simulink model "ej"  (R2017b)
settings: Solver=VariableStepAuto  StartTime=0.0  StopTime=10.0  RelTol=1e-3
settings Model: Creator=Sofia  LastModifiedBy=Sofia

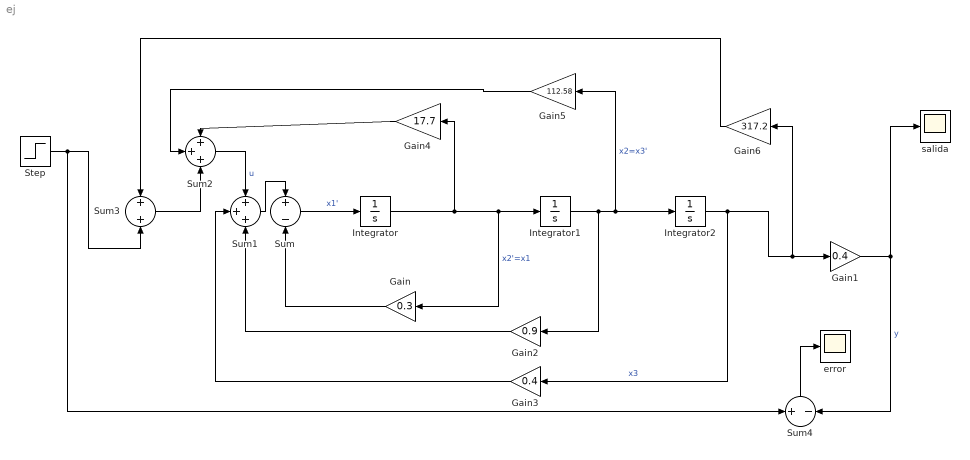
== system ej ==
  Gain : Gain  Gain=0.3
  Gain1 : Gain  Gain=0.4
  Gain2 : Gain  Gain=0.9
  Gain3 : Gain  Gain=0.4
  Gain4 : Gain  Gain=17.7
  Gain5 : Gain  Gain=112.58
  Gain6 : Gain  Gain=317.2
  Integrator : Integrator
  Integrator1 : Integrator
  Integrator2 : Integrator
  Step : Step  SampleTime=0
  Sum : Sum  Inputs=+-
  Sum1 : Sum  Inputs=+++
  Sum2 : Sum  Inputs=+++
  Sum3 : Sum
  Sum4 : Sum  Inputs=+-
  error : Scope
  salida : Scope
  wires:
  Sum/1 -> Integrator/1  "x1'"
  Sum1/1 -> Sum/1
  Integrator/1 -> Gain4/1, Integrator1/1, Gain/1  "x2'=x1"
  Gain/1 -> Sum/2
  Integrator1/1 -> Gain2/1, Gain5/1, Integrator2/1  "x2=x3'"
  Integrator2/1 -> Gain3/1, Gain6/1, Gain1/1  "x3"
  Gain1/1 -> Sum4/2, salida/1  "y"
  Sum2/1 -> Sum1/1  "u"
  Gain2/1 -> Sum1/3
  Gain3/1 -> Sum1/2
  Gain4/1 -> Sum2/1
  Gain5/1 -> Sum2/2
  Sum3/1 -> Sum2/3
  Step/1 -> Sum4/1, Sum3/2
  Gain6/1 -> Sum3/1
  Sum4/1 -> error/1
